simulink model "MCU_Fault"  (R2022b)
settings: Solver=FixedStepDiscrete  StartTime=0.0  StopTime=10.0  FixedStep=1e-4  RelTol=1e-3
values from neighbouring files (symbols this model uses):
  C_Fault_CntDectiontime_u32 = 0.0    [MCU_FaultDiag_Datadictionary.sldd]    (also in MCU_Fault_Datadictionary_objects.m = myPackage.Parameter; MCU_Fault_Datadictionary_objects.sldd)
  C_Fault_IaConfirmCnt_u16 = 0.0    [MCU_FaultDiag_Datadictionary.sldd]    (also in MCU_Fault_Datadictionary_objects.m = myPackage.Parameter; MCU_Fault_Datadictionary_objects.sldd)
  C_Fault_IbConfirmCnt_u16 = 0.0    [MCU_FaultDiag_Datadictionary.sldd]    (also in MCU_Fault_Datadictionary_objects.m = myPackage.Parameter; MCU_Fault_Datadictionary_objects.sldd)
  C_Fault_IbLimit_s32 = 0.0    [MCU_FaultDiag_Datadictionary.sldd]    (also in MCU_Fault_Datadictionary_objects.m = myPackage.Parameter; MCU_Fault_Datadictionary_objects.sldd)
  C_Fault_IcConfirmCnt_u16 = 0.0    [MCU_FaultDiag_Datadictionary.sldd]    (also in MCU_Fault_Datadictionary_objects.m = myPackage.Parameter; MCU_Fault_Datadictionary_objects.sldd)
  C_Fault_IcLimit_s32 = 0.0    [MCU_FaultDiag_Datadictionary.sldd]    (also in MCU_Fault_Datadictionary_objects.m = myPackage.Parameter; MCU_Fault_Datadictionary_objects.sldd)
  C_Fault_IphaseLimitStart_s32 = 0.0    [MCU_FaultDiag_Datadictionary.sldd]    (also in MCU_Fault_Datadictionary_objects.m = myPackage.Parameter; MCU_Fault_Datadictionary_objects.sldd)
  C_Fault_MotorTempSensor_i16 = 0.0    [MCU_FaultDiag_Datadictionary.sldd]    (also in MCU_Fault_Datadictionary_objects.m = myPackage.Parameter; MCU_Fault_Datadictionary_objects.sldd)
  C_Fault_SpdUpFaultConfirmCnt_u16 = 0.0    [MCU_FaultDiag_Datadictionary.sldd]    (also in MCU_Fault_Datadictionary_objects.m = myPackage.Parameter; MCU_Fault_Datadictionary_objects.sldd)
  C_Fault_SpdUpLimitStart_i16 = 0.0    [MCU_FaultDiag_Datadictionary.sldd]    (also in MCU_Fault_Datadictionary_objects.m = myPackage.Parameter; MCU_Fault_Datadictionary_objects.sldd)
  C_Fault_SpdUpLimitStop_i16 = 0.0    [MCU_FaultDiag_Datadictionary.sldd]    (also in MCU_Fault_Datadictionary_objects.m = myPackage.Parameter; MCU_Fault_Datadictionary_objects.sldd)
  C_Fault_SpdUpWarnConfirmCnt_u16 = 0.0    [MCU_FaultDiag_Datadictionary.sldd]    (also in MCU_Fault_Datadictionary_objects.m = myPackage.Parameter; MCU_Fault_Datadictionary_objects.sldd)
  C_Fault_TigbtCircutConfirmCnt_u16 = 0.0    [MCU_FaultDiag_Datadictionary.sldd]    (also in MCU_Fault_Datadictionary_objects.m = myPackage.Parameter; MCU_Fault_Datadictionary_objects.sldd)
  C_Fault_TigbtCircutConfirmTh_u16 = 0.0    [MCU_FaultDiag_Datadictionary.sldd]    (also in MCU_Fault_Datadictionary_objects.m = myPackage.Parameter; MCU_Fault_Datadictionary_objects.sldd)
  C_Fault_TigbtCircutFaultEn_u8 = 0.0    [MCU_FaultDiag_Datadictionary.sldd]    (also in MCU_Fault_Datadictionary_objects.m = myPackage.Parameter; MCU_Fault_Datadictionary_objects.sldd)
  C_Fault_TigbtLimitStart_i16 = 0.0    [MCU_FaultDiag_Datadictionary.sldd]    (also in MCU_Fault_Datadictionary_objects.m = myPackage.Parameter; MCU_Fault_Datadictionary_objects.sldd)
  C_Fault_TigbtLimitStop_i16 = 0.0    [MCU_FaultDiag_Datadictionary.sldd]    (also in MCU_Fault_Datadictionary_objects.m = myPackage.Parameter; MCU_Fault_Datadictionary_objects.sldd)
  C_Fault_TigbtOverConfirmCnt_u16 = 0.0    [MCU_FaultDiag_Datadictionary.sldd]    (also in MCU_Fault_Datadictionary_objects.m = myPackage.Parameter; MCU_Fault_Datadictionary_objects.sldd)
  C_Fault_TigbtWarnConfirmCnt_u16 = 0.0    [MCU_FaultDiag_Datadictionary.sldd]    (also in MCU_Fault_Datadictionary_objects.m = myPackage.Parameter; MCU_Fault_Datadictionary_objects.sldd)
  C_Fault_TmotorCircutConfirmCnt_u16 = 0.0    [MCU_FaultDiag_Datadictionary.sldd]    (also in MCU_Fault_Datadictionary_objects.m = myPackage.Parameter; MCU_Fault_Datadictionary_objects.sldd)
  C_Fault_TmotorCircutConfirmTh_u16 = 0.0    [MCU_FaultDiag_Datadictionary.sldd]    (also in MCU_Fault_Datadictionary_objects.m = myPackage.Parameter; MCU_Fault_Datadictionary_objects.sldd)
  C_Fault_TmotorCircutFaultEn_u8 = 0.0    [MCU_FaultDiag_Datadictionary.sldd]    (also in MCU_Fault_Datadictionary_objects.m = myPackage.Parameter; MCU_Fault_Datadictionary_objects.sldd)
  C_Fault_TmotorLimitStart_i16 = 0.0    [MCU_FaultDiag_Datadictionary.sldd]    (also in MCU_Fault_Datadictionary_objects.m = myPackage.Parameter; MCU_Fault_Datadictionary_objects.sldd)
  C_Fault_TmotorLimitStop_i16 = 0.0    [MCU_FaultDiag_Datadictionary.sldd]    (also in MCU_Fault_Datadictionary_objects.m = myPackage.Parameter; MCU_Fault_Datadictionary_objects.sldd)
  C_Fault_TmotorOverConfirmCnt_u16 = 0.0    [MCU_FaultDiag_Datadictionary.sldd]    (also in MCU_Fault_Datadictionary_objects.m = myPackage.Parameter; MCU_Fault_Datadictionary_objects.sldd)
  C_Fault_TmotorWarnConfirmCnt_u16 = 0.0    [MCU_FaultDiag_Datadictionary.sldd]    (also in MCU_Fault_Datadictionary_objects.m = myPackage.Parameter; MCU_Fault_Datadictionary_objects.sldd)
  C_Fault_UdcLoFaultConfirmCnt_u16 = 0.0    [MCU_FaultDiag_Datadictionary.sldd]    (also in MCU_Fault_Datadictionary_objects.m = myPackage.Parameter; MCU_Fault_Datadictionary_objects.sldd)
  C_Fault_UdcLoWarnConfirmCnt_u16 = 0.0    [MCU_FaultDiag_Datadictionary.sldd]    (also in MCU_Fault_Datadictionary_objects.m = myPackage.Parameter; MCU_Fault_Datadictionary_objects.sldd)
  C_Fault_UdcUpFaultConfirmCnt_u16 = 0.0    [MCU_FaultDiag_Datadictionary.sldd]    (also in MCU_Fault_Datadictionary_objects.m = myPackage.Parameter; MCU_Fault_Datadictionary_objects.sldd)
  C_Fault_UdcUpWarnConfirmCnt_u16 = 0.0    [MCU_FaultDiag_Datadictionary.sldd]    (also in MCU_Fault_Datadictionary_objects.m = myPackage.Parameter; MCU_Fault_Datadictionary_objects.sldd)
undefined symbols (not defined in the file or in its folder): AB_SAMPLE, ABC_SAMPLE, AC_SAMPLE, BC_SAMPLE, ParamCfg_LaValueDefault_u16, ParamCfg_SampleMode_u16, VEHICLE
libraries: simulink x30
(part 2 of 2)

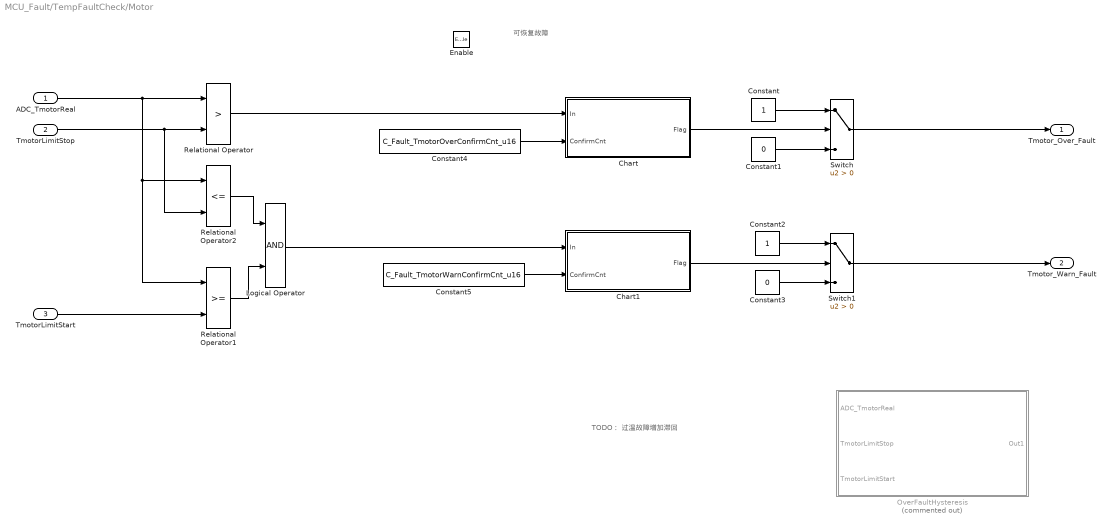
== system MCU_Fault/TempFaultCheck/Motor ==
  note: 可恢复故障
  note: TODO：
      | 过温故障增加滞回
  ADC_TmotorReal : Inport
  TmotorLimitStop : Inport  Port=2
  TmotorLimitStart : Inport  Port=3
  Enable : EnablePort
  Chart : Stateflow chart  TreatAsAtomicUnit=on
  Chart1 : Stateflow chart  TreatAsAtomicUnit=on
  Constant : Constant  OutDataTypeStr=uint32
  Constant1 : Constant  Value=0  OutDataTypeStr=uint32
  Constant2 : Constant  OutDataTypeStr=uint32
  Constant3 : Constant  Value=0  OutDataTypeStr=uint32
  Constant4 : Constant  Value=C_Fault_TmotorOverConfirmCnt_u16
  Constant5 : Constant  Value=C_Fault_TmotorWarnConfirmCnt_u16
  Logical Operator : Logic  AllPortsSameDT=off  OutDataTypeStr=boolean
  "OverFaultHysteresis " : Subsystem  Commented=on
  Relational Operator : RelationalOperator  Operator=>  OutDataTypeStr=boolean  RndMeth=Simplest  InputSameDT=off
  Relational Operator1 : RelationalOperator  OutDataTypeStr=boolean  RndMeth=Simplest  InputSameDT=off
  Relational Operator2 : RelationalOperator  Operator=<=  OutDataTypeStr=boolean  RndMeth=Simplest  InputSameDT=off
  Switch : Switch  Criteria=u2 > Threshold  SaturateOnIntegerOverflow=off  InputSameDT=off
  Switch1 : Switch  Criteria=u2 > Threshold  SaturateOnIntegerOverflow=off  InputSameDT=off
  Tmotor_Over_Fault : Outport
  Tmotor_Warn_Fault : Outport  Port=2
  wires:
  Relational Operator1/1 -> Logical Operator/2
  Constant3/1 -> Switch1/3
  Switch1/1 -> Tmotor_Warn_Fault/1
  Relational Operator2/1 -> Logical Operator/1
  Constant2/1 -> Switch1/1
  Constant1/1 -> Switch/3
  TmotorLimitStart/1 -> Relational Operator1/2
  Constant/1 -> Switch/1
  TmotorLimitStop/1 -> Relational Operator2/2, Relational Operator/2
  Switch/1 -> Tmotor_Over_Fault/1
  ADC_TmotorReal/1 -> Relational Operator2/1, Relational Operator1/1, Relational Operator/1
  Relational Operator/1 -> Chart/1(In)
  Constant4/1 -> Chart/2(ConfirmCnt)
  Chart/1(Flag) -> Switch/2
  Constant5/1 -> Chart1/2(ConfirmCnt)
  Logical Operator/1 -> Chart1/1(In)
  Chart1/1(Flag) -> Switch1/2

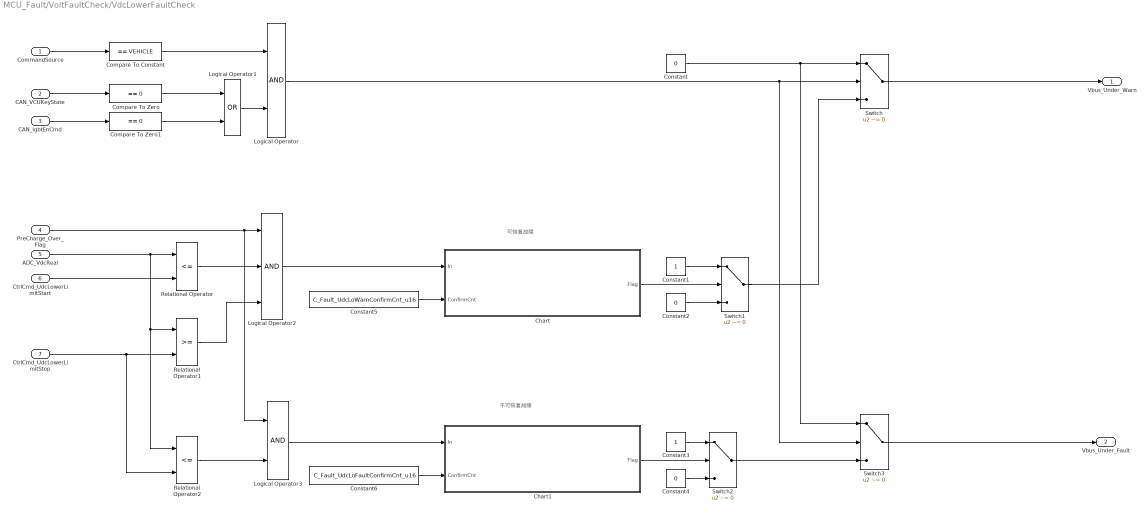
== system MCU_Fault/VoltFaultCheck/VdcLowerFaultCheck ==
  note: 可恢复故障
  note: 不可恢复故障
  CommandSource : Inport
  CAN_VCUKeyState : Inport  Port=2
  CAN_IgbtEnCmd : Inport  Port=3
  PreCharge_Over_Flag : Inport  Port=4
  ADC_VdcReal : Inport  Port=5
  CtrlCmd_UdcLowerLimitStart : Inport  Port=6
  CtrlCmd_UdcLowerLimitStop : Inport  Port=7
  Chart : Stateflow chart  TreatAsAtomicUnit=on
  Chart1 : Stateflow chart  TreatAsAtomicUnit=on
  Compare To Constant : simulink/Logic and Bit Operations/Compare To Constant  relop===  const=VEHICLE  OutDataTypeStr=boolean
  Compare To Zero : simulink/Logic and Bit Operations/Compare To Zero  relop===  OutDataTypeStr=boolean
  Compare To Zero1 : simulink/Logic and Bit Operations/Compare To Zero  relop===  OutDataTypeStr=boolean
  Constant : Constant  Value=0  OutDataTypeStr=uint32
  Constant1 : Constant  OutDataTypeStr=uint32
  Constant2 : Constant  Value=0  OutDataTypeStr=uint32
  Constant3 : Constant  OutDataTypeStr=uint32
  Constant4 : Constant  Value=0  OutDataTypeStr=uint32
  Constant5 : Constant  Value=C_Fault_UdcLoWarnConfirmCnt_u16
  Constant6 : Constant  Value=C_Fault_UdcLoFaultConfirmCnt_u16
  Logical Operator : Logic  AllPortsSameDT=off  OutDataTypeStr=boolean
  Logical Operator1 : Logic  Operator=OR  AllPortsSameDT=off  OutDataTypeStr=boolean
  Logical Operator2 : Logic  Inputs=3  AllPortsSameDT=off  OutDataTypeStr=boolean
  Logical Operator3 : Logic  AllPortsSameDT=off  OutDataTypeStr=boolean
  Relational Operator : RelationalOperator  Operator=<=  OutDataTypeStr=boolean  RndMeth=Simplest  InputSameDT=off
  Relational Operator1 : RelationalOperator  OutDataTypeStr=boolean  RndMeth=Simplest  InputSameDT=off
  Relational Operator2 : RelationalOperator  Operator=<=  OutDataTypeStr=boolean  RndMeth=Simplest  InputSameDT=off
  Switch{,1..3} (4 alike) : Switch  Criteria=u2 ~= 0  SaturateOnIntegerOverflow=off  InputSameDT=off
  Vbus_Under_Warn : Outport
  Vbus_Under_Fault : Outport  Port=2
  wires:
  CommandSource/1 -> Compare To Constant/1
  ADC_VdcReal/1 -> Relational Operator2/1, Relational Operator1/1, Relational Operator/1
  Relational Operator1/1 -> Logical Operator2/3
  Relational Operator2/1 -> Logical Operator3/2
  Constant2/1 -> Switch1/3
  Switch/1 -> Vbus_Under_Warn/1
  Switch1/1 -> Switch/3
  PreCharge_Over_Flag/1 -> Logical Operator3/1, Logical Operator2/1
  CtrlCmd_UdcLowerLimitStop/1 -> Relational Operator2/2, Relational Operator1/2
  Constant3/1 -> Switch2/1
  CAN_IgbtEnCmd/1 -> Compare To Zero1/1
  Constant4/1 -> Switch2/3
  Constant/1 -> Switch3/1, Switch/1
  Relational Operator/1 -> Logical Operator2/2
  Logical Operator/1 -> Switch3/2, Switch/2
  Logical Operator1/1 -> Logical Operator/2
  Compare To Zero/1 -> Logical Operator1/1
  Compare To Zero1/1 -> Logical Operator1/2
  Compare To Constant/1 -> Logical Operator/1
  Constant1/1 -> Switch1/1
  CtrlCmd_UdcLowerLimitStart/1 -> Relational Operator/2
  Switch2/1 -> Switch3/3
  CAN_VCUKeyState/1 -> Compare To Zero/1
  Switch3/1 -> Vbus_Under_Fault/1
  Logical Operator2/1 -> Chart/1(In)
  Chart/1(Flag) -> Switch1/2
  Constant5/1 -> Chart/2(ConfirmCnt)
  Chart1/1(Flag) -> Switch2/2
  Constant6/1 -> Chart1/2(ConfirmCnt)
  Logical Operator3/1 -> Chart1/1(In)

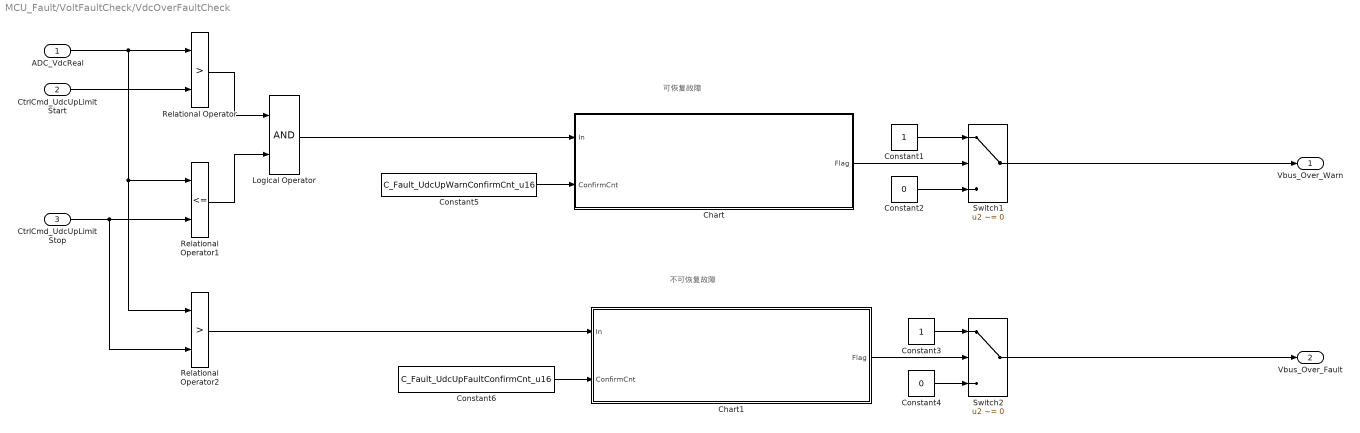
== system MCU_Fault/VoltFaultCheck/VdcOverFaultCheck ==
  note: 可恢复故障
  note: 不可恢复故障
  ADC_VdcReal : Inport
  CtrlCmd_UdcUpLimitStart : Inport  Port=2
  CtrlCmd_UdcUpLimitStop : Inport  Port=3
  Chart : Stateflow chart  TreatAsAtomicUnit=on
  Chart1 : Stateflow chart  TreatAsAtomicUnit=on
  Constant1 : Constant  OutDataTypeStr=uint32
  Constant2 : Constant  Value=0  OutDataTypeStr=uint32
  Constant3 : Constant  OutDataTypeStr=uint32
  Constant4 : Constant  Value=0  OutDataTypeStr=uint32
  Constant5 : Constant  Value=C_Fault_UdcUpWarnConfirmCnt_u16
  Constant6 : Constant  Value=C_Fault_UdcUpFaultConfirmCnt_u16
  Logical Operator : Logic  AllPortsSameDT=off  OutDataTypeStr=boolean
  Relational Operator : RelationalOperator  Operator=>  OutDataTypeStr=boolean  RndMeth=Simplest  InputSameDT=off
  Relational Operator1 : RelationalOperator  Operator=<=  OutDataTypeStr=boolean  RndMeth=Simplest  InputSameDT=off
  Relational Operator2 : RelationalOperator  Operator=>  OutDataTypeStr=boolean  RndMeth=Simplest  InputSameDT=off
  Switch1 : Switch  Criteria=u2 ~= 0  SaturateOnIntegerOverflow=off  InputSameDT=off
  Switch2 : Switch  Criteria=u2 ~= 0  SaturateOnIntegerOverflow=off  InputSameDT=off
  Vbus_Over_Warn : Outport
  Vbus_Over_Fault : Outport  Port=2
  wires:
  CtrlCmd_UdcUpLimitStop/1 -> Relational Operator2/2, Relational Operator1/2
  CtrlCmd_UdcUpLimitStart/1 -> Relational Operator/2
  ADC_VdcReal/1 -> Relational Operator2/1, Relational Operator1/1, Relational Operator/1
  Chart/1(Flag) -> Switch1/2
  Constant1/1 -> Switch1/1
  Constant5/1 -> Chart/2(ConfirmCnt)
  Constant2/1 -> Switch1/3
  Switch1/1 -> Vbus_Over_Warn/1
  Relational Operator1/1 -> Logical Operator/2
  Relational Operator/1 -> Logical Operator/1
  Logical Operator/1 -> Chart/1(In)
  Chart1/1(Flag) -> Switch2/2
  Constant3/1 -> Switch2/1
  Constant6/1 -> Chart1/2(ConfirmCnt)
  Relational Operator2/1 -> Chart1/1(In)
  Constant4/1 -> Switch2/3
  Switch2/1 -> Vbus_Over_Fault/1

== system MCU_Fault/HighTaskFault_100us/InterruptFaultCheck_100us/IaInstantFault ==
  note: 代码里没有Debounce操作，模型里Cnt设置为0，跳过Debounce
  note: 不可恢复故障
  BSW_IaValue : Inport
  Enable : EnablePort
  Chart : Stateflow chart  TreatAsAtomicUnit=on
      settings: RTWSystemCode=Inline
  Constant : Constant  Value=ParamCfg_LaValueDefault_u16
  Constant1 : Constant  Value=C_Fault_IaConfirmCnt_u16  OutDataTypeStr=uint16
  Constant2 : Constant  Value=ParamCfg_LaValueDefault_u16
  Data Type Conversion1 : DataTypeConversion  OutDataTypeStr=uint8  SaturateOnIntegerOverflow=off  RndMeth=Floor
  Gain : Gain  Gain=-1  ParamDataTypeStr=single  OutDataTypeStr=single
  Logical Operator : Logic  Operator=OR  AllPortsSameDT=off  OutDataTypeStr=boolean
  Relational Operator : RelationalOperator  Operator=>  OutDataTypeStr=boolean  RndMeth=Simplest  InputSameDT=off
  Relational Operator1 : RelationalOperator  Operator=<  OutDataTypeStr=boolean  RndMeth=Simplest  InputSameDT=off
  Ia_Instant_Fault : Outport
  wires:
  BSW_IaValue/1 -> Relational Operator1/1, Relational Operator/1  "M_Fault_IaValue_s32"
  Constant/1 -> Gain/1, Relational Operator/2
  Gain/1 -> Relational Operator1/2
  Relational Operator/1 -> Logical Operator/1
  Relational Operator1/1 -> Logical Operator/2
  Chart/1(Flag) -> Ia_Instant_Fault/1
  Logical Operator/1 -> Data Type Conversion1/1
  Constant1/1 -> Chart/2(ConfirmCnt)
  Data Type Conversion1/1 -> Chart/1(In)  "M_Fault_IaInstantFaultNoDeb_u8"

== system MCU_Fault/HighTaskFault_100us/InterruptFaultCheck_100us/IbInstantFault ==
  note: 不可恢复故障
  note: 代码里没有Debounce操作，模型里Cnt设置为0，跳过Debounce
  BSW_IbValue : Inport
  Enable : EnablePort
  Chart : Stateflow chart  TreatAsAtomicUnit=on
  Constant : Constant  Value=C_Fault_IbLimit_s32
  Constant1 : Constant  Value=C_Fault_IbConfirmCnt_u16  OutDataTypeStr=uint16
  Data Type Conversion1 : DataTypeConversion  OutDataTypeStr=uint8  SaturateOnIntegerOverflow=off  RndMeth=Floor
  Gain : Gain  Gain=-1  ParamDataTypeStr=single  OutDataTypeStr=single
  Logical Operator : Logic  Operator=OR  AllPortsSameDT=off  OutDataTypeStr=boolean
  Relational Operator : RelationalOperator  Operator=>  OutDataTypeStr=boolean  RndMeth=Simplest  InputSameDT=off
  Relational Operator1 : RelationalOperator  Operator=<  OutDataTypeStr=boolean  RndMeth=Simplest  InputSameDT=off
  IbInstantFault : Outport
  wires:
  Constant/1 -> Gain/1, Relational Operator/2
  Relational Operator1/1 -> Logical Operator/2
  BSW_IbValue/1 -> Relational Operator1/1, Relational Operator/1  "M_Fault_IbValue_s32"
  Relational Operator/1 -> Logical Operator/1
  Gain/1 -> Relational Operator1/2
  Chart/1(Flag) -> IbInstantFault/1
  Logical Operator/1 -> Data Type Conversion1/1
  Constant1/1 -> Chart/2(ConfirmCnt)
  Data Type Conversion1/1 -> Chart/1(In)  "M_Fault_IbInstantFaultNoDeb_u8"

== system MCU_Fault/HighTaskFault_100us/InterruptFaultCheck_100us/IcInstantFault ==
  note: 不可恢复故障
  note: 代码里没有Debounce操作，模型里Cnt设置为0，跳过Debounce
  BSW_IcValue : Inport
  Enable : EnablePort
  Chart : Stateflow chart  TreatAsAtomicUnit=on
  Constant : Constant  Value=C_Fault_IcLimit_s32
  Constant1 : Constant  Value=C_Fault_IcConfirmCnt_u16  OutDataTypeStr=uint16
  Gain : Gain  Gain=-1  ParamDataTypeStr=single  OutDataTypeStr=single
  Logical Operator : Logic  Operator=OR  AllPortsSameDT=off  OutDataTypeStr=boolean
  Relational Operator : RelationalOperator  Operator=>  OutDataTypeStr=boolean  RndMeth=Simplest  InputSameDT=off
  Relational Operator1 : RelationalOperator  Operator=<  OutDataTypeStr=boolean  RndMeth=Simplest  InputSameDT=off
  IcInstantFault : Outport
  wires:
  BSW_IcValue/1 -> Relational Operator1/1, Relational Operator/1  "M_Fault_IcValue_s32"
  Gain/1 -> Relational Operator1/2
  Relational Operator/1 -> Logical Operator/1
  Constant/1 -> Gain/1, Relational Operator/2
  Logical Operator/1 -> Chart/1(In)
  Relational Operator1/1 -> Logical Operator/2
  Chart/1(Flag) -> IcInstantFault/1
  Constant1/1 -> Chart/2(ConfirmCnt)

== system MCU_Fault/Phase_Fault_Check/Subsystem/IaPhaseFault ==
  ADC_IaValue : Inport
  IphaseLimitStart : Inport  Port=2
  TrqCtrl_TrqCmdFilter : Inport  Port=3
  Enable : EnablePort
  Chart : Stateflow chart  TreatAsAtomicUnit=on
      settings: PortSchema="{\"entries\":[{\"content\":{\"sides\":[{\"content\":{\"connectorIds\":[\"In2\",\"In1\",\"In3\"]},\"type\":\"ConnectorPlacement.EquallySpacedRectSide\",\"uuid\":\"4bd45494-3641-494c-aec0-06e0d93ec36f\"},{\"content\":{\"connectorIds\":[\"Out1\"],\"side\":\"RIGHT\"},\"type\":\"ConnectorPlacement.EquallySpacedRectSide\",\"uuid\":\"b2f4e437-2874-497c-a566-8f2a6ca20672\"},{\"content\":{\"connectorIds\":[],\"side\":\"TOP\"},\"type\":\"ConnectorPlacement.EquallySpacedRectSide\",\"uuid\":\"63e75a5c-0568-4aeb-8607-caa84b5e3a56\"},{\"content\":{\"connectorIds\":[],\"side\":\"BOTTOM\"},\"type\":\"ConnectorPlacement.EquallySpacedRectSide\",\"uuid\":\"5d6ba7e5-7883-4e74-9223-a8682c4d823a\"}]},\"type\":\"ConnectorPlacement.EquallySpacedConnector\",\"uuid\":\"a937fd0f-b134-4493-b942-53644173c4f1\"}],\"packageUris\":[\"http://schema.mathworks.com/mf0/Connector/R2020b\"],\"version\":\"1.0\"}"
  Data Type Conversion : DataTypeConversion  OutDataTypeStr=uint32  SaturateOnIntegerOverflow=off  RndMeth=Floor
  PhaseCurrOverLoad_IaWarn : Outport
  wires:
  ADC_IaValue/1 -> Chart/2(ADC_IaValue)
  IphaseLimitStart/1 -> Chart/1(IphaseLimitStart)
  TrqCtrl_TrqCmdFilter/1 -> Chart/3(TrqCtrl_TrqCmdFilter)
  Chart/1(Flag) -> Data Type Conversion/1
  Data Type Conversion/1 -> PhaseCurrOverLoad_IaWarn/1

== system MCU_Fault/Phase_Fault_Check/Subsystem/IbPhaseFault ==
  ADC_IbValue : Inport
  IphaseLimitStart : Inport  Port=2
  TrqCtrl_TrqCmdFilter : Inport  Port=3
  Enable : EnablePort
  Chart : Stateflow chart  TreatAsAtomicUnit=on
      settings: PortSchema="{\"entries\":[{\"content\":{\"sides\":[{\"content\":{\"connectorIds\":[\"In2\",\"In1\",\"In3\"]},\"type\":\"ConnectorPlacement.EquallySpacedRectSide\",\"uuid\":\"4bd45494-3641-494c-aec0-06e0d93ec36f\"},{\"content\":{\"connectorIds\":[\"Out1\"],\"side\":\"RIGHT\"},\"type\":\"ConnectorPlacement.EquallySpacedRectSide\",\"uuid\":\"b2f4e437-2874-497c-a566-8f2a6ca20672\"},{\"content\":{\"connectorIds\":[],\"side\":\"TOP\"},\"type\":\"ConnectorPlacement.EquallySpacedRectSide\",\"uuid\":\"63e75a5c-0568-4aeb-8607-caa84b5e3a56\"},{\"content\":{\"connectorIds\":[],\"side\":\"BOTTOM\"},\"type\":\"ConnectorPlacement.EquallySpacedRectSide\",\"uuid\":\"5d6ba7e5-7883-4e74-9223-a8682c4d823a\"}]},\"type\":\"ConnectorPlacement.EquallySpacedConnector\",\"uuid\":\"a937fd0f-b134-4493-b942-53644173c4f1\"}],\"packageUris\":[\"http://schema.mathworks.com/mf0/Connector/R2020b\"],\"version\":\"1.0\"}"
  Data Type Conversion : DataTypeConversion  OutDataTypeStr=uint32  SaturateOnIntegerOverflow=off  RndMeth=Floor
  PhaseCurrOverLoad_IbWarn : Outport
  wires:
  Data Type Conversion/1 -> PhaseCurrOverLoad_IbWarn/1
  Chart/1(Flag) -> Data Type Conversion/1
  TrqCtrl_TrqCmdFilter/1 -> Chart/3(TrqCtrl_TrqCmdFilter)
  IphaseLimitStart/1 -> Chart/1(IphaseLimitStart)
  ADC_IbValue/1 -> Chart/2(ADC_IbValue)

== system MCU_Fault/Phase_Fault_Check/Subsystem/IcPhaseFault ==
  ADC_IcValue : Inport
  IphaseLimitStart : Inport  Port=2
  TrqCtrl_TrqCmdFilter : Inport  Port=3
  Enable : EnablePort
  Chart : Stateflow chart  TreatAsAtomicUnit=on
      settings: PortSchema="{\"entries\":[{\"content\":{\"sides\":[{\"content\":{\"connectorIds\":[\"In2\",\"In1\",\"In3\"]},\"type\":\"ConnectorPlacement.EquallySpacedRectSide\",\"uuid\":\"4bd45494-3641-494c-aec0-06e0d93ec36f\"},{\"content\":{\"connectorIds\":[\"Out1\"],\"side\":\"RIGHT\"},\"type\":\"ConnectorPlacement.EquallySpacedRectSide\",\"uuid\":\"b2f4e437-2874-497c-a566-8f2a6ca20672\"},{\"content\":{\"connectorIds\":[],\"side\":\"TOP\"},\"type\":\"ConnectorPlacement.EquallySpacedRectSide\",\"uuid\":\"63e75a5c-0568-4aeb-8607-caa84b5e3a56\"},{\"content\":{\"connectorIds\":[],\"side\":\"BOTTOM\"},\"type\":\"ConnectorPlacement.EquallySpacedRectSide\",\"uuid\":\"5d6ba7e5-7883-4e74-9223-a8682c4d823a\"}]},\"type\":\"ConnectorPlacement.EquallySpacedConnector\",\"uuid\":\"a937fd0f-b134-4493-b942-53644173c4f1\"}],\"packageUris\":[\"http://schema.mathworks.com/mf0/Connector/R2020b\"],\"version\":\"1.0\"}"
  Data Type Conversion : DataTypeConversion  OutDataTypeStr=uint32  SaturateOnIntegerOverflow=off  RndMeth=Floor
  PhaseCurrOverLoad_IcWarn : Outport
  wires:
  ADC_IcValue/1 -> Chart/2(ADC_IcValue)
  IphaseLimitStart/1 -> Chart/1(IphaseLimitStart)
  TrqCtrl_TrqCmdFilter/1 -> Chart/3(TrqCtrl_TrqCmdFilter)
  Chart/1(Flag) -> Data Type Conversion/1
  Data Type Conversion/1 -> PhaseCurrOverLoad_IcWarn/1

== system MCU_Fault/TempFaultCheck/Motor/OverFaultHysteresis  ==
  ADC_TmotorReal : Inport
  TmotorLimitStop : Inport  Port=2
  TmotorLimitStart : Inport  Port=3
  Chart : Stateflow chart  TreatAsAtomicUnit=on
  Chart1 : Stateflow chart  TreatAsAtomicUnit=on
  Constant : Constant  OutDataTypeStr=uint8
  Constant1 : Constant  Value=C_Fault_TmotorOverConfirmCnt_u16
  Constant2 : Constant  Value=0  OutDataTypeStr=uint8
  Constant4 : Constant  Value=C_Fault_TmotorOverConfirmCnt_u16
  Relational Operator : RelationalOperator  Operator=>  OutDataTypeStr=boolean  RndMeth=Simplest  InputSameDT=off
  Relational Operator1 : RelationalOperator  Operator=<  OutDataTypeStr=boolean  RndMeth=Simplest  InputSameDT=off
  Switch : Switch  Criteria=u2 ~= 0  SaturateOnIntegerOverflow=off  InputSameDT=off
  Switch1 : Switch  Criteria=u2 ~= 0  SaturateOnIntegerOverflow=off  InputSameDT=off
  Unit Delay : UnitDelay  SampleTime=-1  HasFrameUpgradeWarning=on
  Out1 : Outport
  wires:
  ADC_TmotorReal/1 -> Relational Operator1/1, Relational Operator/1
  TmotorLimitStop/1 -> Relational Operator/2
  Relational Operator/1 -> Chart/1(In)
  Constant4/1 -> Chart/2(ConfirmCnt)
  Constant/1 -> Switch/1
  Switch/1 -> Out1/1, Unit Delay/1
  TmotorLimitStart/1 -> Relational Operator1/2
  Relational Operator1/1 -> Chart1/1(In)
  Constant1/1 -> Chart1/2(ConfirmCnt)
  Chart1/1(Flag) -> Switch1/2
  Constant2/1 -> Switch1/1
  Chart/1(Flag) -> Switch/2
  Switch1/1 -> Switch/3
  Unit Delay/1 -> Switch1/3

== stateflow chart MCU_Fault/TempFaultCheck/TigbtCircutDebounce ==
  (default) -> (junction 1)
  (junction 1) -> (junction 3) [order 1] : [In >ConfirmTh& En == true]
  (junction 1) -> (junction 13) [order 2] : [En == false]{Flag = (In>ConfirmTh);Cnt = 0}
  (junction 1) -> (junction 13) [order 3] : {Flag = false;
      | Cnt = 0}
  (junction 3) -> (junction 5) : {Cnt = Cnt+1}
  (junction 5) -> (junction 7) [order 1] : [Cnt > ConfirmCnt]
  (junction 5) -> (junction 15) [order 2] : {Flag = false}
  (junction 7) -> (junction 11) : {Flag = true;
      | Cnt = 0}
  (junction 15) -> (junction 13)
  (junction 11) -> (junction 15)
  (junction 13) -> (junction 19)
  data: ConfirmCnt input; In input; ConfirmTh input; Flag output; Cnt local =0; En input

== stateflow chart MCU_Fault/TempFaultCheck/IGBT/Chart ==
  (default) -> (junction 12)
  (junction 12) -> (junction 19) [order 1] : [In == true]
  (junction 12) -> (junction 15) [order 2] : {Flag = false;
      | Cnt = 0;}
  (junction 19) -> (junction 10) : {Cnt = Cnt+1}
  (junction 10) -> (junction 17) [order 1] : [Cnt > ConfirmCnt]
  (junction 10) -> (junction 14) [order 2]
  (junction 17) -> (junction 5) : {Flag = true;
      | Cnt = 0;}
  (junction 14) -> (junction 15)
  (junction 5) -> (junction 14)
  (junction 15) -> (junction 7)
  data: In input; ConfirmCnt input; Flag output =false; Cnt local

== stateflow chart MCU_Fault/TempFaultCheck/IGBT/Chart1 ==
  (default) -> (junction 12)
  (junction 12) -> (junction 19) [order 1] : [In == true]
  (junction 12) -> (junction 15) [order 2] : {Flag = false;
      | Cnt = 0;}
  (junction 19) -> (junction 10) : {Cnt = Cnt+1}
  (junction 10) -> (junction 17) [order 1] : [Cnt > ConfirmCnt]
  (junction 10) -> (junction 14) [order 2]
  (junction 17) -> (junction 5) : {Flag = true;
      | Cnt = 0;}
  (junction 14) -> (junction 15)
  (junction 5) -> (junction 14)
  (junction 15) -> (junction 7)
  data: In input; ConfirmCnt input; Flag output =false; Cnt local

== stateflow chart MCU_Fault/TempFaultCheck/Motor/Chart ==
  (default) -> (junction 12)
  (junction 12) -> (junction 19) [order 1] : [In == true]
  (junction 12) -> (junction 15) [order 2] : {Flag = false;
      | Cnt = 0;}
  (junction 19) -> (junction 10) : {Cnt = Cnt+1}
  (junction 10) -> (junction 17) [order 1] : [Cnt > ConfirmCnt]
  (junction 10) -> (junction 14) [order 2]
  (junction 17) -> (junction 5) : {Flag = true;
      | Cnt = 0;}
  (junction 14) -> (junction 15)
  (junction 5) -> (junction 14)
  (junction 15) -> (junction 7)
  data: In input; ConfirmCnt input; Flag output; Cnt local

== stateflow chart MCU_Fault/TempFaultCheck/Motor/Chart1 ==
  (default) -> (junction 12)
  (junction 12) -> (junction 19) [order 1] : [In == true]
  (junction 12) -> (junction 15) [order 2] : {Flag = false;
      | Cnt = 0;}
  (junction 19) -> (junction 10) : {Cnt = Cnt+1}
  (junction 10) -> (junction 17) [order 1] : [Cnt > ConfirmCnt]
  (junction 10) -> (junction 14) [order 2]
  (junction 17) -> (junction 5) : {Flag = true;
      | Cnt = 0;}
  (junction 14) -> (junction 15)
  (junction 5) -> (junction 14)
  (junction 15) -> (junction 7)
  data: In input; ConfirmCnt input; Flag output; Cnt local

== stateflow chart MCU_Fault/VoltFaultCheck/VdcLowerFaultCheck/Chart ==
  (default) -> (junction 2)
  (junction 2) -> (junction 4) [order 1] : [In == true]
  (junction 2) -> (junction 18) [order 2] : {Flag = false;
      | Cnt = 0}
  (junction 4) -> (junction 6) : {Cnt = Cnt+1}
  (junction 6) -> (junction 11) [order 1] : [Cnt > ConfirmCnt]
  (junction 6) -> (junction 15) [order 2]
  (junction 11) -> (junction 13) : {Flag = true;
      | Cnt = 0;}
  (junction 15) -> (junction 18)
  (junction 13) -> (junction 15)
  (junction 18) -> (junction 21)
  data: In input; Cnt local =0; ConfirmCnt input; Flag output

== stateflow chart MCU_Fault/VoltFaultCheck/VdcLowerFaultCheck/Chart1 ==
  (default) -> (junction 2)
  (junction 2) -> (junction 4) [order 1] : [In == true]
  (junction 2) -> (junction 18) [order 2]
  (junction 4) -> (junction 6) : {Cnt = Cnt+1}
  (junction 6) -> (junction 11) [order 1] : [Cnt > ConfirmCnt]
  (junction 6) -> (junction 15) [order 2]
  (junction 11) -> (junction 13) : {Flag = true;
      | Cnt = 0;}
  (junction 15) -> (junction 18)
  (junction 13) -> (junction 15)
  (junction 18) -> (junction 21)
  data: In input; Cnt local =0; ConfirmCnt input; Flag output

== stateflow chart MCU_Fault/VoltFaultCheck/VdcOverFaultCheck/Chart ==
  (default) -> (junction 2)
  (junction 2) -> (junction 4) [order 1] : [In == true]
  (junction 2) -> (junction 18) [order 2] : {Flag = false;
      | Cnt = 0}
  (junction 4) -> (junction 6) : {Cnt = Cnt+1}
  (junction 6) -> (junction 11) [order 1] : [Cnt > ConfirmCnt]
  (junction 6) -> (junction 15) [order 2]
  (junction 11) -> (junction 13) : {Flag = true;
      | Cnt = 0;}
  (junction 15) -> (junction 18)
  (junction 13) -> (junction 15)
  (junction 18) -> (junction 21)
  data: In input; Cnt local =0; ConfirmCnt input; Flag output

== stateflow chart MCU_Fault/VoltFaultCheck/VdcOverFaultCheck/Chart1 ==
  (default) -> (junction 2)
  (junction 2) -> (junction 4) [order 1] : [In == true]
  (junction 2) -> (junction 18) [order 2]
  (junction 4) -> (junction 6) : {Cnt = Cnt+1}
  (junction 6) -> (junction 11) [order 1] : [Cnt > ConfirmCnt]
  (junction 6) -> (junction 15) [order 2]
  (junction 11) -> (junction 13) : {Flag = true;
      | Cnt = 0;}
  (junction 15) -> (junction 18)
  (junction 13) -> (junction 15)
  (junction 18) -> (junction 21)
  data: In input; Cnt local =0; ConfirmCnt input; Flag output

== stateflow chart MCU_Fault/Speed_Fault_Check/Chart ==
  (default) -> (junction 2)
  (junction 2) -> (junction 4) [order 1] : [In == true]
  (junction 2) -> (junction 18) [order 2] : {Flag = false;
      | Cnt = 0}
  (junction 4) -> (junction 6) : {Cnt = Cnt+1}
  (junction 6) -> (junction 11) [order 1] : [Cnt > ConfirmCnt]
  (junction 6) -> (junction 15) [order 2]
  (junction 11) -> (junction 13) : {Flag = true;
      | Cnt = 0;}
  (junction 15) -> (junction 18)
  (junction 13) -> (junction 15)
  (junction 18) -> (junction 21)
  data: In input; Cnt local =0; ConfirmCnt input; Flag output

== stateflow chart MCU_Fault/Speed_Fault_Check/Chart1 ==
  (default) -> (junction 2)
  (junction 2) -> (junction 4) [order 1] : [In == true]
  (junction 2) -> (junction 18) [order 2]
  (junction 4) -> (junction 6) : {Cnt = Cnt+1}
  (junction 6) -> (junction 11) [order 1] : [Cnt > ConfirmCnt]
  (junction 6) -> (junction 15) [order 2]
  (junction 11) -> (junction 13) : {Flag = true;
      | Cnt = 0;}
  (junction 15) -> (junction 18)
  (junction 13) -> (junction 15)
  (junction 18) -> (junction 21)
  data: In input; Cnt local =0; ConfirmCnt input; Flag output

== stateflow chart MCU_Fault/Phase_Fault_Check/Subsystem/IaPhaseFault/Chart ==
  (default) -> (junction 5)
  (junction 5) -> (junction 7) [order 1] : [ADC_IaValue>IphaseLimitStart || ADC_IaValue<-IphaseLimitStart]
  (junction 5) -> (junction 11) [order 2]
  (junction 7) -> (junction 9) : {Flag = true}
  (junction 11) -> (junction 13) [order 1] : [abs(TrqCtrl_TrqCmdFilter<3)]
  (junction 11) -> (junction 17) [order 2]
  (junction 13) -> (junction 15) : {Flag = false}
  (junction 15) -> (junction 17)
  (junction 9) -> (junction 15)
  (junction 17) -> (junction 21)
  data: IphaseLimitStart input; ADC_IaValue input; TrqCtrl_TrqCmdFilter input; Flag output =false

== stateflow chart MCU_Fault/Phase_Fault_Check/Subsystem/IbPhaseFault/Chart ==
  (default) -> (junction 5)
  (junction 5) -> (junction 7) [order 1] : [ADC_IbValue>IphaseLimitStart || ADC_IbValue<-IphaseLimitStart]
  (junction 5) -> (junction 11) [order 2]
  (junction 7) -> (junction 9) : {Flag = true}
  (junction 11) -> (junction 13) [order 1] : [abs(TrqCtrl_TrqCmdFilter<3)]
  (junction 11) -> (junction 17) [order 2]
  (junction 13) -> (junction 15) : {Flag = false}
  (junction 15) -> (junction 17)
  (junction 9) -> (junction 15)
  (junction 17) -> (junction 21)
  data: IphaseLimitStart input; ADC_IbValue input; TrqCtrl_TrqCmdFilter input; Flag output =false

== stateflow chart MCU_Fault/Phase_Fault_Check/Subsystem/IcPhaseFault/Chart ==
  (default) -> (junction 5)
  (junction 5) -> (junction 7) [order 1] : [ADC_IcValue>IphaseLimitStart || ADC_IcValue<-IphaseLimitStart]
  (junction 5) -> (junction 11) [order 2]
  (junction 7) -> (junction 9) : {Flag = true}
  (junction 11) -> (junction 13) [order 1] : [abs(TrqCtrl_TrqCmdFilter<3)]
  (junction 11) -> (junction 17) [order 2]
  (junction 13) -> (junction 15) : {Flag = false}
  (junction 15) -> (junction 17)
  (junction 9) -> (junction 15)
  (junction 17) -> (junction 21)
  data: IphaseLimitStart input; ADC_IcValue input; TrqCtrl_TrqCmdFilter input; Flag output =false

== stateflow chart MCU_Fault/Lost_Phase_Fault_Check/CurrentDetection/Chart ==
  (default) -> (junction 1) : {LostIaPhase = 0;
      | LostIbPhase = 0;
      | LostIcPhase = 0;}
  (junction 1) -> (junction 6) [order 1] : [Cnt <CntDectionTime]
  (junction 1) -> (junction 18) [order 2] : {IaABSAvg = IaABS/Cnt;
      | IbABSAvg = IbABS/Cnt;
      | IcABSAvg = IcABS/Cnt;}
  (junction 6) -> (junction 10) : {Cnt = Cnt+1;
      | IaABS = IaABS + IaValue;
      | IbABS = IbABS + IbValue;
      | IcABS = IcABS + IcValue}
  (junction 18) -> (junction 23) [order 1] : [IaABSAvg<1]{LostIaPhase = 1}
  (junction 18) -> (junction 30) [order 2]
  (junction 23) -> (junction 25)
  (junction 10) -> (junction 27)
  (junction 25) -> (junction 30)
  (junction 27) -> (junction 25)
  (junction 30) -> (junction 33)
  data: LostIaPhase output; LostIbPhase output; LostIcPhase output; Cnt local =0; CntDectionTime input; IaValue input; IbValue input; IaABS local =0; IbABS local =0; IcABS local =0; IcValue input; IaABSAvg local =0; IbABSAvg local =0; IcABSAvg local

== stateflow chart MCU_Fault/Lost_Phase_Fault_Check/CurrentDetection/Chart1 ==
  (default) -> (junction 1) : {LostIaPhase = 0;
      | LostIbPhase = 0;
      | LostIcPhase = 0;}
  (junction 1) -> (junction 6) [order 1] : [Cnt <CntDectionTime]
  (junction 1) -> (junction 18) [order 2] : {IaABSAvg = IaABS/Cnt;
      | IbABSAvg = IbABS/Cnt;
      | IcABSAvg = IcABS/Cnt;}
  (junction 6) -> (junction 10) : {Cnt = Cnt+1;
      | IaABS = IaABS + IaValue;
      | IbABS = IbABS + IbValue;
      | IcABS = IcABS + IcValue}
  (junction 23) -> (junction 35) [order 1] : [IbABSAvg<1]{LostIbPhase = 1}
  (junction 35) -> (junction 37) [order 1] : [IcABSAvg<1]{LostIcPhase = 1}
  (junction 18) -> (junction 23) [order 1] : [IaABSAvg<1]{LostIaPhase = 1}
  (junction 18) -> (junction 23) [order 2]
  (junction 23) -> (junction 35) [order 2]
  (junction 35) -> (junction 37) [order 2]
  (junction 37) -> (junction 39) : {IaABS = 0;
      | IbABS =0;
      | IcABS=0;}
  (junction 39) -> (junction 64) [order 1] : [(LostIaPhase == 1) || (LostIbPhase == 1) || (LostIcPhase == 1)]{Flag = 1}
  (junction 39) -> (junction 64) [order 2]
  (junction 10) -> (junction 67)
  (junction 67) -> (junction 64)
  (junction 64) -> (junction 70)
  data: LostIaPhase output; LostIbPhase output; LostIcPhase output; Cnt local =0; CntDectionTime input; IaValue input; IbValue input; IaABS local =0; IbABS local =0; IcABS local =0; IcValue input; IaABSAvg local =0; IbABSAvg local =0; IcABSAvg local; Flag output

== stateflow chart MCU_Fault/Lost_Phase_Fault_Check/CurrentDetection/Chart2 ==
  (default) -> (junction 1) [commented out] : {LostIaPhase = 0;
      | LostIbPhase = 0;
      | LostIcPhase = 0;}
  (default) -> (junction 77)
  (junction 1) -> (junction 6) [commented out] : [Cnt <CntDectionTime]
  (junction 1) -> (junction 18) [commented out] : {IaABSAvg = IaABS/Cnt;
      | IbABSAvg = IbABS/Cnt;
      | IcABSAvg = IcABS/Cnt;}
  (junction 6) -> (junction 10) [commented out] : {Cnt = Cnt+1;
      | IaABS = IaABS + IaValue;
      | IbABS = IbABS + IbValue;
      | IcABS = IcABS + IcValue}
  (junction 23) -> (junction 35) [commented out] : [IbABSAvg<1]{LostIbPhase = 1}
  (junction 35) -> (junction 37) [commented out] : [IcABSAvg<1]{LostIcPhase = 1}
  (junction 18) -> (junction 23) [commented out] : [IaABSAvg<1]{LostIaPhase = 1}
  (junction 18) -> (junction 23) [commented out]
  (junction 23) -> (junction 35) [commented out]
  (junction 35) -> (junction 37) [commented out]
  (junction 37) -> (junction 39) [commented out] : {IaABS = 0;
      | IbABS =0;
      | IcABS=0;}
  (junction 39) -> (junction 72) [commented out] : [(LostIaPhase == 1) || (LostIbPhase == 1) || (LostIcPhase == 1)]{Flag = 1}
  (junction 39) -> (junction 72) [commented out]
  (junction 10) -> (junction 67) [commented out]
  (junction 67) -> ? [commented out]
  data: FlagDelay input; LostIaPhase output; LostIbPhase output; LostIcPhase output; Cnt local =0; CntDectionTime input; IaValue input; IbValue input; IaABS local =0; IbABS local =0; IcABS local =0; IcValue input; IaABSAvg local =0; IbABSAvg local =0; IcABSAvg local; Flag output

== stateflow chart MCU_Fault/Lost_Phase_Fault_Check/Enabled Subsystem/Chart ==
  (default) -> (junction 3)
  (junction 3) -> (junction 5) [order 1] : [LossFaultDelay == 0 & Cnt_LowSpd<CntDectionTime]
  (junction 5) -> (junction 11) [order 1] : [Condition == 1]
  (junction 3) -> (junction 9) [order 2] : {Cnt_LowSpd = 0;}
  (junction 5) -> (junction 58) [order 2] : {    IaABSAvg = 0;
      |     IbABSAvg = 0;
      |     IcABSAvg = 0;
      |     IaABS = 0;
      |     IbABS = 0;
      |     IcABS = 0;
      |     Cnt = 0;}
  (junction 11) -> (junction 42) : {Cnt_LowSpd = Cnt_LowSpd + 1}
  (junction 42) -> (junction 27) : {LostIaPhase = 0;
      | LostIbPhase = 0;
      | LostIcPhase = 0;}
  (junction 27) -> (junction 19) [order 1] : [Cnt <CntDectionTime]
  (junction 27) -> (junction 25) [order 2] : {IaABSAvg = IaABS/Cnt;
      | IbABSAvg = IbABS/Cnt;
      | IcABSAvg = IcABS/Cnt;}
  (junction 19) -> (junction 23) : {Cnt = Cnt+1;
      | IaABS = IaABS + IaValue;
      | IbABS = IbABS + IbValue;
      | IcABS = IcABS + IcValue}
  (junction 22) -> (junction 34) [order 1] : [IbABSAvg<1]{LostIbPhase = 1}
  (junction 34) -> (junction 36) [order 1] : [IcABSAvg<1]{LostIcPhase = 1}
  (junction 25) -> (junction 22) [order 1] : [IaABSAvg<1]{LostIaPhase = 1}
  (junction 25) -> (junction 22) [order 2]
  (junction 22) -> (junction 34) [order 2]
  (junction 34) -> (junction 36) [order 2]
  (junction 36) -> (junction 29) : {IaABS = 0;
      | IbABS =0;
      | IcABS=0;}
  (junction 29) -> (junction 31) [order 1] : [(LostIaPhase == 1) || (LostIbPhase == 1) || (LostIcPhase == 1)]{LossPhaseFlag = 1}
  (junction 29) -> (junction 31) [order 2]
  (junction 23) -> (junction 40)
  (junction 40) -> (junction 31)
  (junction 31) -> (junction 39)
  (junction 58) -> (junction 9)
  (junction 39) -> (junction 58)
  (junction 9) -> (junction 62)
  data: LossFaultDelay input; Condition input; CntDectionTime input; Cnt_LowSpd local; IaValue input; IbValue input; IcValue input; Cnt local =0; IaABS local =0; IaABSAvg local =0; IbABS local =0; IbABSAvg local =0; IcABS local =0; IcABSAvg local =0; LostIaPhase output; LostIbPhase output; LostIcPhase output; LossPhaseFlag output

== stateflow chart MCU_Fault/HighTaskFault_100us/InterruptFaultCheck_100us/IaInstantFault/Chart ==
  (default) -> (junction 2)
  (junction 2) -> (junction 4) [order 1] : [In == true]
  (junction 2) -> (junction 18) [order 2] : {Flag = false;
      | Cnt = 0;}
  (junction 4) -> (junction 6) : {Cnt = Cnt+1}
  (junction 6) -> (junction 11) [order 1] : [Cnt > ConfirmCnt]
  (junction 6) -> (junction 15) [order 2]
  (junction 11) -> (junction 13) : {Flag = true;
      | Cnt = 0;}
  (junction 15) -> (junction 18)
  (junction 13) -> (junction 15)
  (junction 18) -> (junction 21)
  data: In input; Cnt local uint16 size=1 =0; ConfirmCnt input; Flag output uint8 =0

== stateflow chart MCU_Fault/HighTaskFault_100us/InterruptFaultCheck_100us/IbInstantFault/Chart ==
  (default) -> (junction 2)
  (junction 2) -> (junction 4) [order 1] : [In == true]
  (junction 2) -> (junction 18) [order 2] : {Flag = false;
      | Cnt = 0;}
  (junction 4) -> (junction 6) : {Cnt = Cnt+1}
  (junction 6) -> (junction 11) [order 1] : [Cnt > ConfirmCnt]
  (junction 6) -> (junction 15) [order 2]
  (junction 11) -> (junction 13) : {Flag = true;
      | Cnt = 0;}
  (junction 15) -> (junction 18)
  (junction 13) -> (junction 15)
  (junction 18) -> (junction 21)
  data: In input; Cnt local uint16 size=1 =0; ConfirmCnt input; Flag output uint8 =0

== stateflow chart MCU_Fault/TempFaultCheck/Motor/OverFaultHysteresis /Chart ==
  (default) -> (junction 12)
  (junction 12) -> (junction 19) [order 1] : [In == true]
  (junction 12) -> (junction 15) [order 2] : {Flag = false;
      | Cnt = 0;}
  (junction 19) -> (junction 10) : {Cnt = Cnt+1}
  (junction 10) -> (junction 17) [order 1] : [Cnt > ConfirmCnt]
  (junction 10) -> (junction 14) [order 2]
  (junction 17) -> (junction 5) : {Flag = true;
      | Cnt = 0;}
  (junction 14) -> (junction 15)
  (junction 5) -> (junction 14)
  (junction 15) -> (junction 7)
  data: In input; ConfirmCnt input; Flag output; Cnt local

== stateflow chart MCU_Fault/TempFaultCheck/Motor/OverFaultHysteresis /Chart1 ==
  (default) -> (junction 12)
  (junction 12) -> (junction 19) [order 1] : [In == true]
  (junction 12) -> (junction 15) [order 2] : {Flag = false;
      | Cnt = 0;}
  (junction 19) -> (junction 10) : {Cnt = Cnt+1}
  (junction 10) -> (junction 17) [order 1] : [Cnt > ConfirmCnt]
  (junction 10) -> (junction 14) [order 2]
  (junction 17) -> (junction 5) : {Flag = true;
      | Cnt = 0;}
  (junction 14) -> (junction 15)
  (junction 5) -> (junction 14)
  (junction 15) -> (junction 7)
  data: In input; ConfirmCnt input; Flag output; Cnt local

== stateflow chart MCU_Fault/HighTaskFault_100us/InterruptFaultCheck_100us/IcInstantFault/Chart ==
  (default) -> (junction 2)
  (junction 2) -> (junction 4) [order 1] : [In == true]
  (junction 2) -> (junction 18) [order 2] : {Flag = false;
      | Cnt = 0;}
  (junction 4) -> (junction 6) : {Cnt = Cnt+1}
  (junction 6) -> (junction 11) [order 1] : [Cnt > ConfirmCnt]
  (junction 6) -> (junction 15) [order 2]
  (junction 11) -> (junction 13) : {Flag = true;
      | Cnt = 0;}
  (junction 15) -> (junction 18)
  (junction 13) -> (junction 15)
  (junction 18) -> (junction 21)
  data: In input; Cnt local uint16 size=1 =0; ConfirmCnt input; Flag output uint8 =0

== stateflow chart MCU_Fault/TempFaultCheck/TmotorDebounce ==
  (default) -> (junction 1)
  (junction 1) -> (junction 3) [order 1] : [In >ConfirmTh& En == true&MotorTempSensor == true]
  (junction 1) -> (junction 13) [order 2] : [En == false]{Flag = (In>ConfirmTh);Cnt = 0}
  (junction 1) -> (junction 13) [order 3] : {Flag = false;
      | Cnt = 0}
  (junction 3) -> (junction 5) : {Cnt = Cnt+1}
  (junction 5) -> (junction 7) [order 1] : [Cnt > ConfirmCnt]
  (junction 5) -> (junction 15) [order 2] : {Flag = false}
  (junction 7) -> (junction 11) : {Flag = true}
  (junction 15) -> (junction 13)
  (junction 11) -> (junction 15)
  (junction 13) -> (junction 19)
  data: ConfirmCnt input; MotorTempSensor input; In input; ConfirmTh input; Flag output; Cnt local =0; En input
